simulink model "test"  (R2015a)
settings: Solver=ode45  StartTime=0.0  StopTime=10.0  RelTol=1e-3
undefined symbols (not defined in the file or in its folder): Afb, Bfb, Cfb, Dfb
libraries: RCTblocks x2
settings Model: Creator=anatole  LastModifiedBy=anatole

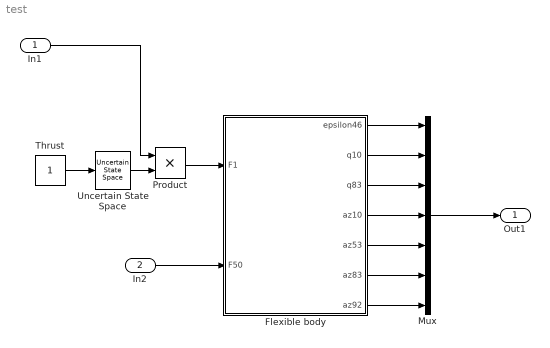
== system test ==
  In1 : Inport
  In2 : Inport  Port=2
  Flexible body : Subsystem
      mask Display:
      | port_label('input',1,'Tail Lateral Force')
      | port_label('input',2,'Fins Lateral Force')
      | 
      | port_label('output',1,'\epsilon_{46}','texmode','on')
      | port_label('output',2,'q_{10}','texmode','on')
      | port_label('output',3,'q_{83}','texmode','on')
      | port_label('output',4,'a_{z10}','texmode','on')
      | port_label('output',5,'a_{z53}','texmode','on')
      | port_label('output',6,'a_{z83}','texmode','on')
      | port_label('output',7,'a_{z92}','texmode','on')
  Mux : Mux  Inputs=7
  Product : Product
  Thrust : Constant
  Uncertain State Space : RCTblocks/Uncertain State Space  Tag=USS  USystem=T0  UValue=[]  X0=[]  uX0=[]
  Out1 : Outport
  wires:
  In2/1 -> Flexible body/2(F50)
  Mux/1 -> Out1/1
  Flexible body/1(epsilon46) -> Mux/1
  Flexible body/2(q10) -> Mux/2
  Flexible body/3(q83) -> Mux/3
  Flexible body/4(az10) -> Mux/4
  Flexible body/5(az53) -> Mux/5
  Flexible body/6(az83) -> Mux/6
  Flexible body/7(az92) -> Mux/7
  Thrust/1 -> Uncertain State Space/1
  In1/1 -> Product/1
  Uncertain State Space/1 -> Product/2
  Product/1 -> Flexible body/1(F1)

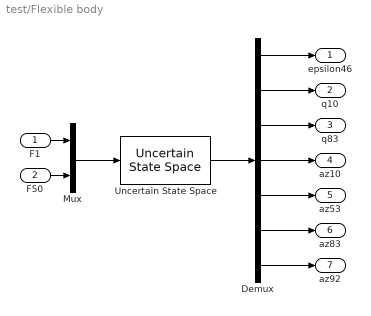
== system test/Flexible body ==
  F1 : Inport
  F50 : Inport  Port=2
  Demux : Demux  Outputs=7
  Mux : Mux  Inputs=2
  Uncertain State Space : RCTblocks/Uncertain State Space  Tag=USS  USystem=ss(Afb,Bfb,Cfb,Dfb)  UValue=[]  X0=[]  uX0=[]
  epsilon46 : Outport
  q10 : Outport  Port=2
  q83 : Outport  Port=3
  az10 : Outport  Port=4
  az53 : Outport  Port=5
  az83 : Outport  Port=6
  az92 : Outport  Port=7
  wires:
  Demux/1 -> epsilon46/1
  Demux/2 -> q10/1
  Demux/3 -> q83/1
  Demux/4 -> az10/1
  Demux/5 -> az53/1
  Demux/6 -> az83/1
  Demux/7 -> az92/1
  F1/1 -> Mux/1
  F50/1 -> Mux/2
  Mux/1 -> Uncertain State Space/1
  Uncertain State Space/1 -> Demux/1
